simulink model "Test_21"  (R2024b)
settings: Solver=FixedStepAuto  StartTime=0.0  StopTime=50  RelTol=1e-3
undefined symbols (not defined in the file): BOOL, DINT, OTL, slplc
libraries: arduinolib x4
(part 9 of 10)

== matlab function Test_21/PLC Controller Suite/__Logic/Task/Program/__Logic/XIC1/__Format ==
  data: BlockEnable input; RungIn input; RungOut input; data input
function setBlockFormat(BlockEnable, RungIn, RungOut, data)

if data~=0 && data~=1
    error('slplc:inivalidBooleanValue', 'Invalid boolean value %d', data);
end
data = logical(data);

% set parent block colors
coder.extrinsic('slplc.utils.setBlockAppearance');
persistent lastBlockEnable lastRungIn lastRungOut lastData isInit lastAnimation lastDataShow;
if isempty(lastBlockEnable)
    lastBlockEnable = true;
end
if isempty(lastRungIn)
    lastRungIn = false;
end
if isempty(lastRungOut)
    lastRungOut = false;
end
if isempty(lastData)
    lastData = data;
end
if isempty(isInit)
    isInit = true;
else
    isInit = false;
end
if isempty(lastAnimation)
    lastAnimation = false;
end
if isempty(lastDataShow)
    lastDataShow = false;
end

[animation, dataShow] = slplc.utils.setBlockAppearance('set', '%<PLCOperandTag>', {}, {}, ...
    ' = ', {'ForegroundColor'}, ...
    isInit,  ...
    BlockEnable, lastBlockEnable, ...
    RungIn,  lastRungIn, ...
    RungOut, lastRungOut, ...
    data, lastData, ...
    lastAnimation, lastDataShow);

lastBlockEnable = BlockEnable;
lastRungIn      = RungIn;
lastRungOut     = RungOut;
lastData        = data;
lastAnimation   = animation;
lastDataShow    = dataShow;
end

== matlab function Test_21/PLC Controller Suite/__Logic/Task/Program/__Logic/Junction/__Format ==
  data: BlockEnable input; RungOut input
function setBlockFormat(BlockEnable, RungOut)
% set parent block colors
coder.extrinsic('slplc.utils.setBlockAppearance');
persistent lastBlockEnable isInit lastRungOut lastAnimation lastRungOutShow;
if isempty(lastBlockEnable)
    lastBlockEnable = true;
end

if isempty(isInit)
    isInit = true;
else
    isInit = false;
end

if isempty(lastRungOut)
    lastRungOut = RungOut;
end

if isempty(lastAnimation)
    lastAnimation = false;
end

if isempty(lastRungOutShow)
    lastRungOutShow = false;
end

[animation, dataShow] = slplc.utils.setBlockAppearance('set', '', {'black', 'black'}, {}, ...
    '', {'ForegroundColor', 'BackgroundColor'}, ...
    isInit,  ...
    BlockEnable, lastBlockEnable, ...
    RungOut,   lastRungOut, ...
    RungOut,   lastRungOut, ...
    [],    [], ...
    lastAnimation, lastRungOutShow);

lastBlockEnable     = BlockEnable;
lastRungOut         = RungOut;
lastAnimation       = animation;
lastRungOutShow     = dataShow;
end

== matlab function Test_21/PLC Controller Suite/__Logic/Task/Program/__Logic/OTL4/__Format ==
  data: BlockEnable input; RungIn input; RungOut input; data input
function setBlockFormat(BlockEnable, RungIn, RungOut, data)

if data~=0 && data~=1
    error('slplc:inivalidBooleanValue', 'Invalid boolean value %d', data);
end
data = logical(data);

% set parent block colors
coder.extrinsic('slplc.utils.setBlockAppearance');
persistent lastBlockEnable lastRungIn lastRungOut lastData isInit lastAnimation lastDataShow;
if isempty(lastBlockEnable)
    lastBlockEnable = true;
end
if isempty(lastRungIn)
    lastRungIn = false;
end
if isempty(lastRungOut)
    lastRungOut = false;
end
if isempty(lastData)
    lastData = data;
end
if isempty(isInit)
    isInit = true;
else
    isInit = false;
end
if isempty(lastAnimation)
    lastAnimation = false;
end
if isempty(lastDataShow)
    lastDataShow = false;
end

[animation, dataShow] = slplc.utils.setBlockAppearance('set', '%<PLCOperandTag>', {}, {}, ...
    ' = ', {'ForegroundColor'}, ...
    isInit,  ...
    BlockEnable, lastBlockEnable, ...
    RungIn,  lastRungIn, ...
    RungOut, lastRungOut, ...
    data, lastData, ...
    lastAnimation, lastDataShow);

lastBlockEnable = BlockEnable;
lastRungIn      = RungIn;
lastRungOut     = RungOut;
lastData        = data;
lastAnimation   = animation;
lastDataShow    = dataShow;
end

== matlab function Test_21/PLC Controller Suite/__Logic/Task/Program/__Logic/XIC3/__Format ==
  data: BlockEnable input; RungIn input; RungOut input; data input
function setBlockFormat(BlockEnable, RungIn, RungOut, data)

if data~=0 && data~=1
    error('slplc:inivalidBooleanValue', 'Invalid boolean value %d', data);
end
data = logical(data);

% set parent block colors
coder.extrinsic('slplc.utils.setBlockAppearance');
persistent lastBlockEnable lastRungIn lastRungOut lastData isInit lastAnimation lastDataShow;
if isempty(lastBlockEnable)
    lastBlockEnable = true;
end
if isempty(lastRungIn)
    lastRungIn = false;
end
if isempty(lastRungOut)
    lastRungOut = false;
end
if isempty(lastData)
    lastData = data;
end
if isempty(isInit)
    isInit = true;
else
    isInit = false;
end
if isempty(lastAnimation)
    lastAnimation = false;
end
if isempty(lastDataShow)
    lastDataShow = false;
end

[animation, dataShow] = slplc.utils.setBlockAppearance('set', '%<PLCOperandTag>', {}, {}, ...
    ' = ', {'ForegroundColor'}, ...
    isInit,  ...
    BlockEnable, lastBlockEnable, ...
    RungIn,  lastRungIn, ...
    RungOut, lastRungOut, ...
    data, lastData, ...
    lastAnimation, lastDataShow);

lastBlockEnable = BlockEnable;
lastRungIn      = RungIn;
lastRungOut     = RungOut;
lastData        = data;
lastAnimation   = animation;
lastDataShow    = dataShow;
end

== matlab function Test_21/PLC Controller Suite/__Logic/Task/Program/__Logic/OTL1/__Format ==
  data: BlockEnable input; RungIn input; RungOut input; data input
function setBlockFormat(BlockEnable, RungIn, RungOut, data)

if data~=0 && data~=1
    error('slplc:inivalidBooleanValue', 'Invalid boolean value %d', data);
end
data = logical(data);

% set parent block colors
coder.extrinsic('slplc.utils.setBlockAppearance');
persistent lastBlockEnable lastRungIn lastRungOut lastData isInit lastAnimation lastDataShow;
if isempty(lastBlockEnable)
    lastBlockEnable = true;
end
if isempty(lastRungIn)
    lastRungIn = false;
end
if isempty(lastRungOut)
    lastRungOut = false;
end
if isempty(lastData)
    lastData = data;
end
if isempty(isInit)
    isInit = true;
else
    isInit = false;
end
if isempty(lastAnimation)
    lastAnimation = false;
end
if isempty(lastDataShow)
    lastDataShow = false;
end

[animation, dataShow] = slplc.utils.setBlockAppearance('set', '%<PLCOperandTag>', {}, {}, ...
    ' = ', {'ForegroundColor'}, ...
    isInit,  ...
    BlockEnable, lastBlockEnable, ...
    RungIn,  lastRungIn, ...
    RungOut, lastRungOut, ...
    data, lastData, ...
    lastAnimation, lastDataShow);

lastBlockEnable = BlockEnable;
lastRungIn      = RungIn;
lastRungOut     = RungOut;
lastData        = data;
lastAnimation   = animation;
lastDataShow    = dataShow;
end

== matlab function Test_21/PLC Controller Suite/__Logic/Task/Program/__Logic/OTU9/__Format ==
  data: BlockEnable input; RungIn input; RungOut input; data input
function setBlockFormat(BlockEnable, RungIn, RungOut, data)

if data~=0 && data~=1
    error('slplc:inivalidBooleanValue', 'Invalid boolean value %d', data);
end
data = logical(data);

% set parent block colors
coder.extrinsic('slplc.utils.setBlockAppearance');
persistent lastBlockEnable lastRungIn lastRungOut lastData isInit lastAnimation lastDataShow;
if isempty(lastBlockEnable)
    lastBlockEnable = true;
end
if isempty(lastRungIn)
    lastRungIn = false;
end
if isempty(lastRungOut)
    lastRungOut = false;
end
if isempty(lastData)
    lastData = data;
end
if isempty(isInit)
    isInit = true;
else
    isInit = false;
end
if isempty(lastAnimation)
    lastAnimation = false;
end
if isempty(lastDataShow)
    lastDataShow = false;
end

[animation, dataShow] = slplc.utils.setBlockAppearance('set', '%<PLCOperandTag>', {}, {}, ...
    ' = ', {'ForegroundColor'}, ...
    isInit,  ...
    BlockEnable, lastBlockEnable, ...
    RungIn,  lastRungIn, ...
    RungOut, lastRungOut, ...
    data, lastData, ...
    lastAnimation, lastDataShow);

lastBlockEnable = BlockEnable;
lastRungIn      = RungIn;
lastRungOut     = RungOut;
lastData        = data;
lastAnimation   = animation;
lastDataShow    = dataShow;
end

== matlab function Test_21/PLC Controller Suite/__Logic/Task/Program/__Logic/OTU3/__Format ==
  data: BlockEnable input; RungIn input; RungOut input; data input
function setBlockFormat(BlockEnable, RungIn, RungOut, data)

if data~=0 && data~=1
    error('slplc:inivalidBooleanValue', 'Invalid boolean value %d', data);
end
data = logical(data);

% set parent block colors
coder.extrinsic('slplc.utils.setBlockAppearance');
persistent lastBlockEnable lastRungIn lastRungOut lastData isInit lastAnimation lastDataShow;
if isempty(lastBlockEnable)
    lastBlockEnable = true;
end
if isempty(lastRungIn)
    lastRungIn = false;
end
if isempty(lastRungOut)
    lastRungOut = false;
end
if isempty(lastData)
    lastData = data;
end
if isempty(isInit)
    isInit = true;
else
    isInit = false;
end
if isempty(lastAnimation)
    lastAnimation = false;
end
if isempty(lastDataShow)
    lastDataShow = false;
end

[animation, dataShow] = slplc.utils.setBlockAppearance('set', '%<PLCOperandTag>', {}, {}, ...
    ' = ', {'ForegroundColor'}, ...
    isInit,  ...
    BlockEnable, lastBlockEnable, ...
    RungIn,  lastRungIn, ...
    RungOut, lastRungOut, ...
    data, lastData, ...
    lastAnimation, lastDataShow);

lastBlockEnable = BlockEnable;
lastRungIn      = RungIn;
lastRungOut     = RungOut;
lastData        = data;
lastAnimation   = animation;
lastDataShow    = dataShow;
end

== matlab function Test_21/PLC Controller Suite/__Logic/Task/Program/__Logic/OTU4/__Format ==
  data: BlockEnable input; RungIn input; RungOut input; data input
function setBlockFormat(BlockEnable, RungIn, RungOut, data)

if data~=0 && data~=1
    error('slplc:inivalidBooleanValue', 'Invalid boolean value %d', data);
end
data = logical(data);

% set parent block colors
coder.extrinsic('slplc.utils.setBlockAppearance');
persistent lastBlockEnable lastRungIn lastRungOut lastData isInit lastAnimation lastDataShow;
if isempty(lastBlockEnable)
    lastBlockEnable = true;
end
if isempty(lastRungIn)
    lastRungIn = false;
end
if isempty(lastRungOut)
    lastRungOut = false;
end
if isempty(lastData)
    lastData = data;
end
if isempty(isInit)
    isInit = true;
else
    isInit = false;
end
if isempty(lastAnimation)
    lastAnimation = false;
end
if isempty(lastDataShow)
    lastDataShow = false;
end

[animation, dataShow] = slplc.utils.setBlockAppearance('set', '%<PLCOperandTag>', {}, {}, ...
    ' = ', {'ForegroundColor'}, ...
    isInit,  ...
    BlockEnable, lastBlockEnable, ...
    RungIn,  lastRungIn, ...
    RungOut, lastRungOut, ...
    data, lastData, ...
    lastAnimation, lastDataShow);

lastBlockEnable = BlockEnable;
lastRungIn      = RungIn;
lastRungOut     = RungOut;
lastData        = data;
lastAnimation   = animation;
lastDataShow    = dataShow;
end

== matlab function Test_21/PLC Controller Suite/__Logic/Task/Program/__Logic/OTL7/__Format ==
  data: BlockEnable input; RungIn input; RungOut input; data input
function setBlockFormat(BlockEnable, RungIn, RungOut, data)

if data~=0 && data~=1
    error('slplc:inivalidBooleanValue', 'Invalid boolean value %d', data);
end
data = logical(data);

% set parent block colors
coder.extrinsic('slplc.utils.setBlockAppearance');
persistent lastBlockEnable lastRungIn lastRungOut lastData isInit lastAnimation lastDataShow;
if isempty(lastBlockEnable)
    lastBlockEnable = true;
end
if isempty(lastRungIn)
    lastRungIn = false;
end
if isempty(lastRungOut)
    lastRungOut = false;
end
if isempty(lastData)
    lastData = data;
end
if isempty(isInit)
    isInit = true;
else
    isInit = false;
end
if isempty(lastAnimation)
    lastAnimation = false;
end
if isempty(lastDataShow)
    lastDataShow = false;
end

[animation, dataShow] = slplc.utils.setBlockAppearance('set', '%<PLCOperandTag>', {}, {}, ...
    ' = ', {'ForegroundColor'}, ...
    isInit,  ...
    BlockEnable, lastBlockEnable, ...
    RungIn,  lastRungIn, ...
    RungOut, lastRungOut, ...
    data, lastData, ...
    lastAnimation, lastDataShow);

lastBlockEnable = BlockEnable;
lastRungIn      = RungIn;
lastRungOut     = RungOut;
lastData        = data;
lastAnimation   = animation;
lastDataShow    = dataShow;
end

== matlab function Test_21/PLC Controller Suite/__Logic/Task/Program/__Logic/TON/Instruction_Enable/__Logic ==
  data: EN output; TT output; RungIn input; PRE input; EN input; DN input; DN output; ACC output; ACC input; currentTime input; lastTime input
function [EN, TT, DN, ACC]  = TON(RungIn, PRE, EN, DN, ACC, currentTime, lastTime)
% TON algorithm

if RungIn
    % Rung-condition-in is True
    if PRE < 0 || ACC < 0
        error('slplc:TONError', '.PRE or .ACC cannot be negtive values');
    end
    TT = true;
    if ~DN
        if EN
            deltaT = currentTime - lastTime;
            ACC = ACC + cast(deltaT, class(ACC));
            if ACC == intmax(class(ACC)) || ACC >= PRE
                TT = false;
                DN = true;
            end
        end
    else
        TT = false;
    end
    EN = true;
    % True end
else
    % Rung-condition-in is False
    EN    = false;
    TT    = false;
    DN    = false;
    ACC   = cast(0, class(ACC));
    % False end
end

end

== matlab function Test_21/PLC Controller Suite/__Logic/Task/Program/__Logic/XIC10/__Format ==
  data: BlockEnable input; RungIn input; RungOut input; data input
function setBlockFormat(BlockEnable, RungIn, RungOut, data)

if data~=0 && data~=1
    error('slplc:inivalidBooleanValue', 'Invalid boolean value %d', data);
end
data = logical(data);

% set parent block colors
coder.extrinsic('slplc.utils.setBlockAppearance');
persistent lastBlockEnable lastRungIn lastRungOut lastData isInit lastAnimation lastDataShow;
if isempty(lastBlockEnable)
    lastBlockEnable = true;
end
if isempty(lastRungIn)
    lastRungIn = false;
end
if isempty(lastRungOut)
    lastRungOut = false;
end
if isempty(lastData)
    lastData = data;
end
if isempty(isInit)
    isInit = true;
else
    isInit = false;
end
if isempty(lastAnimation)
    lastAnimation = false;
end
if isempty(lastDataShow)
    lastDataShow = false;
end

[animation, dataShow] = slplc.utils.setBlockAppearance('set', '%<PLCOperandTag>', {}, {}, ...
    ' = ', {'ForegroundColor'}, ...
    isInit,  ...
    BlockEnable, lastBlockEnable, ...
    RungIn,  lastRungIn, ...
    RungOut, lastRungOut, ...
    data, lastData, ...
    lastAnimation, lastDataShow);

lastBlockEnable = BlockEnable;
lastRungIn      = RungIn;
lastRungOut     = RungOut;
lastData        = data;
lastAnimation   = animation;
lastDataShow    = dataShow;
end

== matlab function Test_21/PLC Controller Suite/__Logic/Task/Program/__Logic/OTU2/__Format ==
  data: BlockEnable input; RungIn input; RungOut input; data input
function setBlockFormat(BlockEnable, RungIn, RungOut, data)

if data~=0 && data~=1
    error('slplc:inivalidBooleanValue', 'Invalid boolean value %d', data);
end
data = logical(data);

% set parent block colors
coder.extrinsic('slplc.utils.setBlockAppearance');
persistent lastBlockEnable lastRungIn lastRungOut lastData isInit lastAnimation lastDataShow;
if isempty(lastBlockEnable)
    lastBlockEnable = true;
end
if isempty(lastRungIn)
    lastRungIn = false;
end
if isempty(lastRungOut)
    lastRungOut = false;
end
if isempty(lastData)
    lastData = data;
end
if isempty(isInit)
    isInit = true;
else
    isInit = false;
end
if isempty(lastAnimation)
    lastAnimation = false;
end
if isempty(lastDataShow)
    lastDataShow = false;
end

[animation, dataShow] = slplc.utils.setBlockAppearance('set', '%<PLCOperandTag>', {}, {}, ...
    ' = ', {'ForegroundColor'}, ...
    isInit,  ...
    BlockEnable, lastBlockEnable, ...
    RungIn,  lastRungIn, ...
    RungOut, lastRungOut, ...
    data, lastData, ...
    lastAnimation, lastDataShow);

lastBlockEnable = BlockEnable;
lastRungIn      = RungIn;
lastRungOut     = RungOut;
lastData        = data;
lastAnimation   = animation;
lastDataShow    = dataShow;
end

== matlab function Test_21/PLC Controller Suite/__Logic/Task/Program/__Logic/XIO/__Format ==
  data: BlockEnable input; RungIn input; RungOut input; data input
function setBlockFormat(BlockEnable, RungIn, RungOut, data)

if data~=0 && data~=1
    error('slplc:inivalidBooleanValue', 'Invalid boolean value %d', data);
end
data = logical(data);

% set parent block colors
coder.extrinsic('slplc.utils.setBlockAppearance');
persistent lastBlockEnable lastRungIn lastRungOut lastData isInit lastAnimation lastDataShow;
if isempty(lastBlockEnable)
    lastBlockEnable = true;
end
if isempty(lastRungIn)
    lastRungIn = false;
end
if isempty(lastRungOut)
    lastRungOut = false;
end
if isempty(lastData)
    lastData = data;
end
if isempty(isInit)
    isInit = true;
else
    isInit = false;
end
if isempty(lastAnimation)
    lastAnimation = false;
end
if isempty(lastDataShow)
    lastDataShow = false;
end

[animation, dataShow] = slplc.utils.setBlockAppearance('set', '%<PLCOperandTag>', {}, {}, ...
    ' = ', {'ForegroundColor'}, ...
    isInit,  ...
    BlockEnable, lastBlockEnable, ...
    RungIn,  lastRungIn, ...
    RungOut, lastRungOut, ...
    data, lastData, ...
    lastAnimation, lastDataShow);

lastBlockEnable = BlockEnable;
lastRungIn      = RungIn;
lastRungOut     = RungOut;
lastData        = data;
lastAnimation   = animation;
lastDataShow    = dataShow;
end

== matlab function Test_21/PLC Controller Suite/__Logic/Task/Program/__Logic/XIC8/__Format ==
  data: BlockEnable input; RungIn input; RungOut input; data input
function setBlockFormat(BlockEnable, RungIn, RungOut, data)

if data~=0 && data~=1
    error('slplc:inivalidBooleanValue', 'Invalid boolean value %d', data);
end
data = logical(data);

% set parent block colors
coder.extrinsic('slplc.utils.setBlockAppearance');
persistent lastBlockEnable lastRungIn lastRungOut lastData isInit lastAnimation lastDataShow;
if isempty(lastBlockEnable)
    lastBlockEnable = true;
end
if isempty(lastRungIn)
    lastRungIn = false;
end
if isempty(lastRungOut)
    lastRungOut = false;
end
if isempty(lastData)
    lastData = data;
end
if isempty(isInit)
    isInit = true;
else
    isInit = false;
end
if isempty(lastAnimation)
    lastAnimation = false;
end
if isempty(lastDataShow)
    lastDataShow = false;
end

[animation, dataShow] = slplc.utils.setBlockAppearance('set', '%<PLCOperandTag>', {}, {}, ...
    ' = ', {'ForegroundColor'}, ...
    isInit,  ...
    BlockEnable, lastBlockEnable, ...
    RungIn,  lastRungIn, ...
    RungOut, lastRungOut, ...
    data, lastData, ...
    lastAnimation, lastDataShow);

lastBlockEnable = BlockEnable;
lastRungIn      = RungIn;
lastRungOut     = RungOut;
lastData        = data;
lastAnimation   = animation;
lastDataShow    = dataShow;
end

== matlab function Test_21/PLC Controller Suite/__Logic/Task/Program/__Logic/XIC6/__Format ==
  data: BlockEnable input; RungIn input; RungOut input; data input
function setBlockFormat(BlockEnable, RungIn, RungOut, data)

if data~=0 && data~=1
    error('slplc:inivalidBooleanValue', 'Invalid boolean value %d', data);
end
data = logical(data);

% set parent block colors
coder.extrinsic('slplc.utils.setBlockAppearance');
persistent lastBlockEnable lastRungIn lastRungOut lastData isInit lastAnimation lastDataShow;
if isempty(lastBlockEnable)
    lastBlockEnable = true;
end
if isempty(lastRungIn)
    lastRungIn = false;
end
if isempty(lastRungOut)
    lastRungOut = false;
end
if isempty(lastData)
    lastData = data;
end
if isempty(isInit)
    isInit = true;
else
    isInit = false;
end
if isempty(lastAnimation)
    lastAnimation = false;
end
if isempty(lastDataShow)
    lastDataShow = false;
end

[animation, dataShow] = slplc.utils.setBlockAppearance('set', '%<PLCOperandTag>', {}, {}, ...
    ' = ', {'ForegroundColor'}, ...
    isInit,  ...
    BlockEnable, lastBlockEnable, ...
    RungIn,  lastRungIn, ...
    RungOut, lastRungOut, ...
    data, lastData, ...
    lastAnimation, lastDataShow);

lastBlockEnable = BlockEnable;
lastRungIn      = RungIn;
lastRungOut     = RungOut;
lastData        = data;
lastAnimation   = animation;
lastDataShow    = dataShow;
end

== matlab function Test_21/PLC Controller Suite/__Logic/Task/Program/__Logic/OTU10/__Format ==
  data: BlockEnable input; RungIn input; RungOut input; data input
function setBlockFormat(BlockEnable, RungIn, RungOut, data)

if data~=0 && data~=1
    error('slplc:inivalidBooleanValue', 'Invalid boolean value %d', data);
end
data = logical(data);

% set parent block colors
coder.extrinsic('slplc.utils.setBlockAppearance');
persistent lastBlockEnable lastRungIn lastRungOut lastData isInit lastAnimation lastDataShow;
if isempty(lastBlockEnable)
    lastBlockEnable = true;
end
if isempty(lastRungIn)
    lastRungIn = false;
end
if isempty(lastRungOut)
    lastRungOut = false;
end
if isempty(lastData)
    lastData = data;
end
if isempty(isInit)
    isInit = true;
else
    isInit = false;
end
if isempty(lastAnimation)
    lastAnimation = false;
end
if isempty(lastDataShow)
    lastDataShow = false;
end

[animation, dataShow] = slplc.utils.setBlockAppearance('set', '%<PLCOperandTag>', {}, {}, ...
    ' = ', {'ForegroundColor'}, ...
    isInit,  ...
    BlockEnable, lastBlockEnable, ...
    RungIn,  lastRungIn, ...
    RungOut, lastRungOut, ...
    data, lastData, ...
    lastAnimation, lastDataShow);

lastBlockEnable = BlockEnable;
lastRungIn      = RungIn;
lastRungOut     = RungOut;
lastData        = data;
lastAnimation   = animation;
lastDataShow    = dataShow;
end

== matlab function Test_21/PLC Controller Suite/__Logic/Task/Program/__Logic/OTL2/__Format ==
  data: BlockEnable input; RungIn input; RungOut input; data input
function setBlockFormat(BlockEnable, RungIn, RungOut, data)

if data~=0 && data~=1
    error('slplc:inivalidBooleanValue', 'Invalid boolean value %d', data);
end
data = logical(data);

% set parent block colors
coder.extrinsic('slplc.utils.setBlockAppearance');
persistent lastBlockEnable lastRungIn lastRungOut lastData isInit lastAnimation lastDataShow;
if isempty(lastBlockEnable)
    lastBlockEnable = true;
end
if isempty(lastRungIn)
    lastRungIn = false;
end
if isempty(lastRungOut)
    lastRungOut = false;
end
if isempty(lastData)
    lastData = data;
end
if isempty(isInit)
    isInit = true;
else
    isInit = false;
end
if isempty(lastAnimation)
    lastAnimation = false;
end
if isempty(lastDataShow)
    lastDataShow = false;
end

[animation, dataShow] = slplc.utils.setBlockAppearance('set', '%<PLCOperandTag>', {}, {}, ...
    ' = ', {'ForegroundColor'}, ...
    isInit,  ...
    BlockEnable, lastBlockEnable, ...
    RungIn,  lastRungIn, ...
    RungOut, lastRungOut, ...
    data, lastData, ...
    lastAnimation, lastDataShow);

lastBlockEnable = BlockEnable;
lastRungIn      = RungIn;
lastRungOut     = RungOut;
lastData        = data;
lastAnimation   = animation;
lastDataShow    = dataShow;
end

== matlab function Test_21/PLC Controller Suite/__Logic/Task/Program/__Logic/OTU/__Format ==
  data: BlockEnable input; RungIn input; RungOut input; data input
function setBlockFormat(BlockEnable, RungIn, RungOut, data)

if data~=0 && data~=1
    error('slplc:inivalidBooleanValue', 'Invalid boolean value %d', data);
end
data = logical(data);

% set parent block colors
coder.extrinsic('slplc.utils.setBlockAppearance');
persistent lastBlockEnable lastRungIn lastRungOut lastData isInit lastAnimation lastDataShow;
if isempty(lastBlockEnable)
    lastBlockEnable = true;
end
if isempty(lastRungIn)
    lastRungIn = false;
end
if isempty(lastRungOut)
    lastRungOut = false;
end
if isempty(lastData)
    lastData = data;
end
if isempty(isInit)
    isInit = true;
else
    isInit = false;
end
if isempty(lastAnimation)
    lastAnimation = false;
end
if isempty(lastDataShow)
    lastDataShow = false;
end

[animation, dataShow] = slplc.utils.setBlockAppearance('set', '%<PLCOperandTag>', {}, {}, ...
    ' = ', {'ForegroundColor'}, ...
    isInit,  ...
    BlockEnable, lastBlockEnable, ...
    RungIn,  lastRungIn, ...
    RungOut, lastRungOut, ...
    data, lastData, ...
    lastAnimation, lastDataShow);

lastBlockEnable = BlockEnable;
lastRungIn      = RungIn;
lastRungOut     = RungOut;
lastData        = data;
lastAnimation   = animation;
lastDataShow    = dataShow;
end

== matlab function Test_21/PLC Controller Suite/__Logic/Task/Program/__Logic/OTU1/__Format ==
  data: BlockEnable input; RungIn input; RungOut input; data input
function setBlockFormat(BlockEnable, RungIn, RungOut, data)

if data~=0 && data~=1
    error('slplc:inivalidBooleanValue', 'Invalid boolean value %d', data);
end
data = logical(data);

% set parent block colors
coder.extrinsic('slplc.utils.setBlockAppearance');
persistent lastBlockEnable lastRungIn lastRungOut lastData isInit lastAnimation lastDataShow;
if isempty(lastBlockEnable)
    lastBlockEnable = true;
end
if isempty(lastRungIn)
    lastRungIn = false;
end
if isempty(lastRungOut)
    lastRungOut = false;
end
if isempty(lastData)
    lastData = data;
end
if isempty(isInit)
    isInit = true;
else
    isInit = false;
end
if isempty(lastAnimation)
    lastAnimation = false;
end
if isempty(lastDataShow)
    lastDataShow = false;
end

[animation, dataShow] = slplc.utils.setBlockAppearance('set', '%<PLCOperandTag>', {}, {}, ...
    ' = ', {'ForegroundColor'}, ...
    isInit,  ...
    BlockEnable, lastBlockEnable, ...
    RungIn,  lastRungIn, ...
    RungOut, lastRungOut, ...
    data, lastData, ...
    lastAnimation, lastDataShow);

lastBlockEnable = BlockEnable;
lastRungIn      = RungIn;
lastRungOut     = RungOut;
lastData        = data;
lastAnimation   = animation;
lastDataShow    = dataShow;
end

== matlab function Test_21/PLC Controller Suite/__Logic/Task/Program/__Logic/XIO3/__Format ==
  data: BlockEnable input; RungIn input; RungOut input; data input
function setBlockFormat(BlockEnable, RungIn, RungOut, data)

if data~=0 && data~=1
    error('slplc:inivalidBooleanValue', 'Invalid boolean value %d', data);
end
data = logical(data);

% set parent block colors
coder.extrinsic('slplc.utils.setBlockAppearance');
persistent lastBlockEnable lastRungIn lastRungOut lastData isInit lastAnimation lastDataShow;
if isempty(lastBlockEnable)
    lastBlockEnable = true;
end
if isempty(lastRungIn)
    lastRungIn = false;
end
if isempty(lastRungOut)
    lastRungOut = false;
end
if isempty(lastData)
    lastData = data;
end
if isempty(isInit)
    isInit = true;
else
    isInit = false;
end
if isempty(lastAnimation)
    lastAnimation = false;
end
if isempty(lastDataShow)
    lastDataShow = false;
end

[animation, dataShow] = slplc.utils.setBlockAppearance('set', '%<PLCOperandTag>', {}, {}, ...
    ' = ', {'ForegroundColor'}, ...
    isInit,  ...
    BlockEnable, lastBlockEnable, ...
    RungIn,  lastRungIn, ...
    RungOut, lastRungOut, ...
    data, lastData, ...
    lastAnimation, lastDataShow);

lastBlockEnable = BlockEnable;
lastRungIn      = RungIn;
lastRungOut     = RungOut;
lastData        = data;
lastAnimation   = animation;
lastDataShow    = dataShow;
end

== matlab function Test_21/PLC Controller Suite/__Logic/Task/Program/__Logic/OTU5/__Format ==
  data: BlockEnable input; RungIn input; RungOut input; data input
function setBlockFormat(BlockEnable, RungIn, RungOut, data)

if data~=0 && data~=1
    error('slplc:inivalidBooleanValue', 'Invalid boolean value %d', data);
end
data = logical(data);

% set parent block colors
coder.extrinsic('slplc.utils.setBlockAppearance');
persistent lastBlockEnable lastRungIn lastRungOut lastData isInit lastAnimation lastDataShow;
if isempty(lastBlockEnable)
    lastBlockEnable = true;
end
if isempty(lastRungIn)
    lastRungIn = false;
end
if isempty(lastRungOut)
    lastRungOut = false;
end
if isempty(lastData)
    lastData = data;
end
if isempty(isInit)
    isInit = true;
else
    isInit = false;
end
if isempty(lastAnimation)
    lastAnimation = false;
end
if isempty(lastDataShow)
    lastDataShow = false;
end

[animation, dataShow] = slplc.utils.setBlockAppearance('set', '%<PLCOperandTag>', {}, {}, ...
    ' = ', {'ForegroundColor'}, ...
    isInit,  ...
    BlockEnable, lastBlockEnable, ...
    RungIn,  lastRungIn, ...
    RungOut, lastRungOut, ...
    data, lastData, ...
    lastAnimation, lastDataShow);

lastBlockEnable = BlockEnable;
lastRungIn      = RungIn;
lastRungOut     = RungOut;
lastData        = data;
lastAnimation   = animation;
lastDataShow    = dataShow;
end

== matlab function Test_21/PLC Controller Suite/__Logic/Task/Program/__Logic/XIC7/__Format ==
  data: BlockEnable input; RungIn input; RungOut input; data input
function setBlockFormat(BlockEnable, RungIn, RungOut, data)

if data~=0 && data~=1
    error('slplc:inivalidBooleanValue', 'Invalid boolean value %d', data);
end
data = logical(data);

% set parent block colors
coder.extrinsic('slplc.utils.setBlockAppearance');
persistent lastBlockEnable lastRungIn lastRungOut lastData isInit lastAnimation lastDataShow;
if isempty(lastBlockEnable)
    lastBlockEnable = true;
end
if isempty(lastRungIn)
    lastRungIn = false;
end
if isempty(lastRungOut)
    lastRungOut = false;
end
if isempty(lastData)
    lastData = data;
end
if isempty(isInit)
    isInit = true;
else
    isInit = false;
end
if isempty(lastAnimation)
    lastAnimation = false;
end
if isempty(lastDataShow)
    lastDataShow = false;
end

[animation, dataShow] = slplc.utils.setBlockAppearance('set', '%<PLCOperandTag>', {}, {}, ...
    ' = ', {'ForegroundColor'}, ...
    isInit,  ...
    BlockEnable, lastBlockEnable, ...
    RungIn,  lastRungIn, ...
    RungOut, lastRungOut, ...
    data, lastData, ...
    lastAnimation, lastDataShow);

lastBlockEnable = BlockEnable;
lastRungIn      = RungIn;
lastRungOut     = RungOut;
lastData        = data;
lastAnimation   = animation;
lastDataShow    = dataShow;
end

== matlab function Test_21/PLC Controller Suite/__Logic/Task/Program/__Logic/XIO2/__Format ==
  data: BlockEnable input; RungIn input; RungOut input; data input
function setBlockFormat(BlockEnable, RungIn, RungOut, data)

if data~=0 && data~=1
    error('slplc:inivalidBooleanValue', 'Invalid boolean value %d', data);
end
data = logical(data);

% set parent block colors
coder.extrinsic('slplc.utils.setBlockAppearance');
persistent lastBlockEnable lastRungIn lastRungOut lastData isInit lastAnimation lastDataShow;
if isempty(lastBlockEnable)
    lastBlockEnable = true;
end
if isempty(lastRungIn)
    lastRungIn = false;
end
if isempty(lastRungOut)
    lastRungOut = false;
end
if isempty(lastData)
    lastData = data;
end
if isempty(isInit)
    isInit = true;
else
    isInit = false;
end
if isempty(lastAnimation)
    lastAnimation = false;
end
if isempty(lastDataShow)
    lastDataShow = false;
end

[animation, dataShow] = slplc.utils.setBlockAppearance('set', '%<PLCOperandTag>', {}, {}, ...
    ' = ', {'ForegroundColor'}, ...
    isInit,  ...
    BlockEnable, lastBlockEnable, ...
    RungIn,  lastRungIn, ...
    RungOut, lastRungOut, ...
    data, lastData, ...
    lastAnimation, lastDataShow);

lastBlockEnable = BlockEnable;
lastRungIn      = RungIn;
lastRungOut     = RungOut;
lastData        = data;
lastAnimation   = animation;
lastDataShow    = dataShow;
end

== matlab function Test_21/PLC Controller Suite/__Logic/Task/Program/__Logic/OTE3/__Format ==
  data: BlockEnable input; RungIn input; RungOut input; data input
function setBlockFormat(BlockEnable, RungIn, RungOut, data)

if data~=0 && data~=1
    error('slplc:inivalidBooleanValue', 'Invalid boolean value %d', data);
end
data = logical(data);

% set parent block colors
coder.extrinsic('slplc.utils.setBlockAppearance');
persistent lastBlockEnable lastRungIn lastRungOut lastData isInit lastAnimation lastDataShow;
if isempty(lastBlockEnable)
    lastBlockEnable = true;
end
if isempty(lastRungIn)
    lastRungIn = false;
end
if isempty(lastRungOut)
    lastRungOut = false;
end
if isempty(lastData)
    lastData = data;
end
if isempty(isInit)
    isInit = true;
else
    isInit = false;
end
if isempty(lastAnimation)
    lastAnimation = false;
end
if isempty(lastDataShow)
    lastDataShow = false;
end

[animation, dataShow] = slplc.utils.setBlockAppearance('set', '%<PLCOperandTag>', {}, {}, ...
    ' = ', {'ForegroundColor'}, ...
    isInit,  ...
    BlockEnable, lastBlockEnable, ...
    RungIn,  lastRungIn, ...
    RungOut, lastRungOut, ...
    data, lastData, ...
    lastAnimation, lastDataShow);

lastBlockEnable = BlockEnable;
lastRungIn      = RungIn;
lastRungOut     = RungOut;
lastData        = data;
lastAnimation   = animation;
lastDataShow    = dataShow;
end

== matlab function Test_21/PLC Controller Suite/__Logic/Task/Program/__Logic/TON3/Instruction_Enable/__Logic ==
  data: EN output; TT output; RungIn input; PRE input; EN input; DN input; DN output; ACC output; ACC input; currentTime input; lastTime input
function [EN, TT, DN, ACC]  = TON(RungIn, PRE, EN, DN, ACC, currentTime, lastTime)
% TON algorithm

if RungIn
    % Rung-condition-in is True
    if PRE < 0 || ACC < 0
        error('slplc:TONError', '.PRE or .ACC cannot be negtive values');
    end
    TT = true;
    if ~DN
        if EN
            deltaT = currentTime - lastTime;
            ACC = ACC + cast(deltaT, class(ACC));
            if ACC == intmax(class(ACC)) || ACC >= PRE
                TT = false;
                DN = true;
            end
        end
    else
        TT = false;
    end
    EN = true;
    % True end
else
    % Rung-condition-in is False
    EN    = false;
    TT    = false;
    DN    = false;
    ACC   = cast(0, class(ACC));
    % False end
end

end

== matlab function Test_21/PLC Controller Suite/__Logic/Task/Program/__Logic/TON3/__Format ==
  data: BlockEnable input; RungIn input; RungOut input; data input
function setBlockFormat(BlockEnable, RungIn, RungOut, data)
% set parent block colors
coder.extrinsic('slplc.utils.setBlockAppearance');
persistent lastBlockEnable lastRungIn lastRungOut lastData isInit lastAnimation lastDataShow;
if isempty(lastBlockEnable)
    lastBlockEnable = true;
end
if isempty(lastRungIn)
    lastRungIn = false;
end
if isempty(lastRungOut)
    lastRungOut = false;
end
if isempty(lastData)
    lastData = data;
end
if isempty(isInit)
    isInit = true;
else
    isInit = false;
end
if isempty(lastAnimation)
    lastAnimation = false;
end
if isempty(lastDataShow)
    lastDataShow = false;
end

[animation, dataShow] = slplc.utils.setBlockAppearance('set', '%<PLCBlockType>: %<PLCOperandTag>', {}, {}, ...
    ' = ', {'ForegroundColor'}, ...
    isInit,  ...
    BlockEnable, lastBlockEnable, ...
    RungIn,  lastRungIn, ...
    RungOut, lastRungOut, ...
    data, lastData, ...
    lastAnimation, lastDataShow);

lastBlockEnable = BlockEnable;
lastRungIn      = RungIn;
lastRungOut     = RungOut;
lastData        = data;
lastAnimation   = animation;
lastDataShow    = dataShow;
end

== matlab function Test_21/PLC Controller Suite/__Logic/Task/Program/__Logic/OTU6/__Format ==
  data: BlockEnable input; RungIn input; RungOut input; data input
function setBlockFormat(BlockEnable, RungIn, RungOut, data)

if data~=0 && data~=1
    error('slplc:inivalidBooleanValue', 'Invalid boolean value %d', data);
end
data = logical(data);

% set parent block colors
coder.extrinsic('slplc.utils.setBlockAppearance');
persistent lastBlockEnable lastRungIn lastRungOut lastData isInit lastAnimation lastDataShow;
if isempty(lastBlockEnable)
    lastBlockEnable = true;
end
if isempty(lastRungIn)
    lastRungIn = false;
end
if isempty(lastRungOut)
    lastRungOut = false;
end
if isempty(lastData)
    lastData = data;
end
if isempty(isInit)
    isInit = true;
else
    isInit = false;
end
if isempty(lastAnimation)
    lastAnimation = false;
end
if isempty(lastDataShow)
    lastDataShow = false;
end

[animation, dataShow] = slplc.utils.setBlockAppearance('set', '%<PLCOperandTag>', {}, {}, ...
    ' = ', {'ForegroundColor'}, ...
    isInit,  ...
    BlockEnable, lastBlockEnable, ...
    RungIn,  lastRungIn, ...
    RungOut, lastRungOut, ...
    data, lastData, ...
    lastAnimation, lastDataShow);

lastBlockEnable = BlockEnable;
lastRungIn      = RungIn;
lastRungOut     = RungOut;
lastData        = data;
lastAnimation   = animation;
lastDataShow    = dataShow;
end

== matlab function Test_21/PLC Controller Suite/__Logic/Task/Program/__Logic/XIC9/__Format ==
  data: BlockEnable input; RungIn input; RungOut input; data input
function setBlockFormat(BlockEnable, RungIn, RungOut, data)

if data~=0 && data~=1
    error('slplc:inivalidBooleanValue', 'Invalid boolean value %d', data);
end
data = logical(data);

% set parent block colors
coder.extrinsic('slplc.utils.setBlockAppearance');
persistent lastBlockEnable lastRungIn lastRungOut lastData isInit lastAnimation lastDataShow;
if isempty(lastBlockEnable)
    lastBlockEnable = true;
end
if isempty(lastRungIn)
    lastRungIn = false;
end
if isempty(lastRungOut)
    lastRungOut = false;
end
if isempty(lastData)
    lastData = data;
end
if isempty(isInit)
    isInit = true;
else
    isInit = false;
end
if isempty(lastAnimation)
    lastAnimation = false;
end
if isempty(lastDataShow)
    lastDataShow = false;
end

[animation, dataShow] = slplc.utils.setBlockAppearance('set', '%<PLCOperandTag>', {}, {}, ...
    ' = ', {'ForegroundColor'}, ...
    isInit,  ...
    BlockEnable, lastBlockEnable, ...
    RungIn,  lastRungIn, ...
    RungOut, lastRungOut, ...
    data, lastData, ...
    lastAnimation, lastDataShow);

lastBlockEnable = BlockEnable;
lastRungIn      = RungIn;
lastRungOut     = RungOut;
lastData        = data;
lastAnimation   = animation;
lastDataShow    = dataShow;
end

== matlab function Test_21/PLC Controller Suite/__Logic/Task/Program/__Logic/Junction1/__Format ==
  data: BlockEnable input; RungOut input
function setBlockFormat(BlockEnable, RungOut)
% set parent block colors
coder.extrinsic('slplc.utils.setBlockAppearance');
persistent lastBlockEnable isInit lastRungOut lastAnimation lastRungOutShow;
if isempty(lastBlockEnable)
    lastBlockEnable = true;
end

if isempty(isInit)
    isInit = true;
else
    isInit = false;
end

if isempty(lastRungOut)
    lastRungOut = RungOut;
end

if isempty(lastAnimation)
    lastAnimation = false;
end

if isempty(lastRungOutShow)
    lastRungOutShow = false;
end

[animation, dataShow] = slplc.utils.setBlockAppearance('set', '', {'black', 'black'}, {}, ...
    '', {'ForegroundColor', 'BackgroundColor'}, ...
    isInit,  ...
    BlockEnable, lastBlockEnable, ...
    RungOut,   lastRungOut, ...
    RungOut,   lastRungOut, ...
    [],    [], ...
    lastAnimation, lastRungOutShow);

lastBlockEnable     = BlockEnable;
lastRungOut         = RungOut;
lastAnimation       = animation;
lastRungOutShow     = dataShow;
end

== matlab function Test_21/PLC Controller Suite/__Logic/Task/Program/__Logic/OTU7/__Format ==
  data: BlockEnable input; RungIn input; RungOut input; data input
function setBlockFormat(BlockEnable, RungIn, RungOut, data)

if data~=0 && data~=1
    error('slplc:inivalidBooleanValue', 'Invalid boolean value %d', data);
end
data = logical(data);

% set parent block colors
coder.extrinsic('slplc.utils.setBlockAppearance');
persistent lastBlockEnable lastRungIn lastRungOut lastData isInit lastAnimation lastDataShow;
if isempty(lastBlockEnable)
    lastBlockEnable = true;
end
if isempty(lastRungIn)
    lastRungIn = false;
end
if isempty(lastRungOut)
    lastRungOut = false;
end
if isempty(lastData)
    lastData = data;
end
if isempty(isInit)
    isInit = true;
else
    isInit = false;
end
if isempty(lastAnimation)
    lastAnimation = false;
end
if isempty(lastDataShow)
    lastDataShow = false;
end

[animation, dataShow] = slplc.utils.setBlockAppearance('set', '%<PLCOperandTag>', {}, {}, ...
    ' = ', {'ForegroundColor'}, ...
    isInit,  ...
    BlockEnable, lastBlockEnable, ...
    RungIn,  lastRungIn, ...
    RungOut, lastRungOut, ...
    data, lastData, ...
    lastAnimation, lastDataShow);

lastBlockEnable = BlockEnable;
lastRungIn      = RungIn;
lastRungOut     = RungOut;
lastData        = data;
lastAnimation   = animation;
lastDataShow    = dataShow;
end

== matlab function Test_21/PLC Controller Suite/__Logic/Task/Program/__Logic/OTL5/__Format ==
  data: BlockEnable input; RungIn input; RungOut input; data input
function setBlockFormat(BlockEnable, RungIn, RungOut, data)

if data~=0 && data~=1
    error('slplc:inivalidBooleanValue', 'Invalid boolean value %d', data);
end
data = logical(data);

% set parent block colors
coder.extrinsic('slplc.utils.setBlockAppearance');
persistent lastBlockEnable lastRungIn lastRungOut lastData isInit lastAnimation lastDataShow;
if isempty(lastBlockEnable)
    lastBlockEnable = true;
end
if isempty(lastRungIn)
    lastRungIn = false;
end
if isempty(lastRungOut)
    lastRungOut = false;
end
if isempty(lastData)
    lastData = data;
end
if isempty(isInit)
    isInit = true;
else
    isInit = false;
end
if isempty(lastAnimation)
    lastAnimation = false;
end
if isempty(lastDataShow)
    lastDataShow = false;
end

[animation, dataShow] = slplc.utils.setBlockAppearance('set', '%<PLCOperandTag>', {}, {}, ...
    ' = ', {'ForegroundColor'}, ...
    isInit,  ...
    BlockEnable, lastBlockEnable, ...
    RungIn,  lastRungIn, ...
    RungOut, lastRungOut, ...
    data, lastData, ...
    lastAnimation, lastDataShow);

lastBlockEnable = BlockEnable;
lastRungIn      = RungIn;
lastRungOut     = RungOut;
lastData        = data;
lastAnimation   = animation;
lastDataShow    = dataShow;
end

== matlab function Test_21/PLC Controller Suite/__Logic/Task/Program/__Logic/OTL6/__Format ==
  data: BlockEnable input; RungIn input; RungOut input; data input
function setBlockFormat(BlockEnable, RungIn, RungOut, data)

if data~=0 && data~=1
    error('slplc:inivalidBooleanValue', 'Invalid boolean value %d', data);
end
data = logical(data);

% set parent block colors
coder.extrinsic('slplc.utils.setBlockAppearance');
persistent lastBlockEnable lastRungIn lastRungOut lastData isInit lastAnimation lastDataShow;
if isempty(lastBlockEnable)
    lastBlockEnable = true;
end
if isempty(lastRungIn)
    lastRungIn = false;
end
if isempty(lastRungOut)
    lastRungOut = false;
end
if isempty(lastData)
    lastData = data;
end
if isempty(isInit)
    isInit = true;
else
    isInit = false;
end
if isempty(lastAnimation)
    lastAnimation = false;
end
if isempty(lastDataShow)
    lastDataShow = false;
end

[animation, dataShow] = slplc.utils.setBlockAppearance('set', '%<PLCOperandTag>', {}, {}, ...
    ' = ', {'ForegroundColor'}, ...
    isInit,  ...
    BlockEnable, lastBlockEnable, ...
    RungIn,  lastRungIn, ...
    RungOut, lastRungOut, ...
    data, lastData, ...
    lastAnimation, lastDataShow);

lastBlockEnable = BlockEnable;
lastRungIn      = RungIn;
lastRungOut     = RungOut;
lastData        = data;
lastAnimation   = animation;
lastDataShow    = dataShow;
end

== matlab function Test_21/PLC Controller Suite/__Logic/Task/Program/__Logic/XIO1/__Format ==
  data: BlockEnable input; RungIn input; RungOut input; data input
function setBlockFormat(BlockEnable, RungIn, RungOut, data)

if data~=0 && data~=1
    error('slplc:inivalidBooleanValue', 'Invalid boolean value %d', data);
end
data = logical(data);

% set parent block colors
coder.extrinsic('slplc.utils.setBlockAppearance');
persistent lastBlockEnable lastRungIn lastRungOut lastData isInit lastAnimation lastDataShow;
if isempty(lastBlockEnable)
    lastBlockEnable = true;
end
if isempty(lastRungIn)
    lastRungIn = false;
end
if isempty(lastRungOut)
    lastRungOut = false;
end
if isempty(lastData)
    lastData = data;
end
if isempty(isInit)
    isInit = true;
else
    isInit = false;
end
if isempty(lastAnimation)
    lastAnimation = false;
end
if isempty(lastDataShow)
    lastDataShow = false;
end

[animation, dataShow] = slplc.utils.setBlockAppearance('set', '%<PLCOperandTag>', {}, {}, ...
    ' = ', {'ForegroundColor'}, ...
    isInit,  ...
    BlockEnable, lastBlockEnable, ...
    RungIn,  lastRungIn, ...
    RungOut, lastRungOut, ...
    data, lastData, ...
    lastAnimation, lastDataShow);

lastBlockEnable = BlockEnable;
lastRungIn      = RungIn;
lastRungOut     = RungOut;
lastData        = data;
lastAnimation   = animation;
lastDataShow    = dataShow;
end

== matlab function Test_21/PLC Controller Suite/__Logic/Task/Program/__Logic/OTU8/__Format ==
  data: BlockEnable input; RungIn input; RungOut input; data input
function setBlockFormat(BlockEnable, RungIn, RungOut, data)

if data~=0 && data~=1
    error('slplc:inivalidBooleanValue', 'Invalid boolean value %d', data);
end
data = logical(data);

% set parent block colors
coder.extrinsic('slplc.utils.setBlockAppearance');
persistent lastBlockEnable lastRungIn lastRungOut lastData isInit lastAnimation lastDataShow;
if isempty(lastBlockEnable)
    lastBlockEnable = true;
end
if isempty(lastRungIn)
    lastRungIn = false;
end
if isempty(lastRungOut)
    lastRungOut = false;
end
if isempty(lastData)
    lastData = data;
end
if isempty(isInit)
    isInit = true;
else
    isInit = false;
end
if isempty(lastAnimation)
    lastAnimation = false;
end
if isempty(lastDataShow)
    lastDataShow = false;
end

[animation, dataShow] = slplc.utils.setBlockAppearance('set', '%<PLCOperandTag>', {}, {}, ...
    ' = ', {'ForegroundColor'}, ...
    isInit,  ...
    BlockEnable, lastBlockEnable, ...
    RungIn,  lastRungIn, ...
    RungOut, lastRungOut, ...
    data, lastData, ...
    lastAnimation, lastDataShow);

lastBlockEnable = BlockEnable;
lastRungIn      = RungIn;
lastRungOut     = RungOut;
lastData        = data;
lastAnimation   = animation;
lastDataShow    = dataShow;
end

== matlab function Test_21/PLC Controller Suite/__Logic/Task/Program/__Logic/OTE4/__Format ==
  data: BlockEnable input; RungIn input; RungOut input; data input
function setBlockFormat(BlockEnable, RungIn, RungOut, data)

if data~=0 && data~=1
    error('slplc:inivalidBooleanValue', 'Invalid boolean value %d', data);
end
data = logical(data);

% set parent block colors
coder.extrinsic('slplc.utils.setBlockAppearance');
persistent lastBlockEnable lastRungIn lastRungOut lastData isInit lastAnimation lastDataShow;
if isempty(lastBlockEnable)
    lastBlockEnable = true;
end
if isempty(lastRungIn)
    lastRungIn = false;
end
if isempty(lastRungOut)
    lastRungOut = false;
end
if isempty(lastData)
    lastData = data;
end
if isempty(isInit)
    isInit = true;
else
    isInit = false;
end
if isempty(lastAnimation)
    lastAnimation = false;
end
if isempty(lastDataShow)
    lastDataShow = false;
end

[animation, dataShow] = slplc.utils.setBlockAppearance('set', '%<PLCOperandTag>', {}, {}, ...
    ' = ', {'ForegroundColor'}, ...
    isInit,  ...
    BlockEnable, lastBlockEnable, ...
    RungIn,  lastRungIn, ...
    RungOut, lastRungOut, ...
    data, lastData, ...
    lastAnimation, lastDataShow);

lastBlockEnable = BlockEnable;
lastRungIn      = RungIn;
lastRungOut     = RungOut;
lastData        = data;
lastAnimation   = animation;
lastDataShow    = dataShow;
end

== matlab function Test_21/PLC Controller Suite/__Logic/Task/Program/__Logic/TON4/Instruction_Enable/__Logic ==
  data: EN output; TT output; RungIn input; PRE input; EN input; DN input; DN output; ACC output; ACC input; currentTime input; lastTime input
function [EN, TT, DN, ACC]  = TON(RungIn, PRE, EN, DN, ACC, currentTime, lastTime)
% TON algorithm

if RungIn
    % Rung-condition-in is True
    if PRE < 0 || ACC < 0
        error('slplc:TONError', '.PRE or .ACC cannot be negtive values');
    end
    TT = true;
    if ~DN
        if EN
            deltaT = currentTime - lastTime;
            ACC = ACC + cast(deltaT, class(ACC));
            if ACC == intmax(class(ACC)) || ACC >= PRE
                TT = false;
                DN = true;
            end
        end
    else
        TT = false;
    end
    EN = true;
    % True end
else
    % Rung-condition-in is False
    EN    = false;
    TT    = false;
    DN    = false;
    ACC   = cast(0, class(ACC));
    % False end
end

end

== matlab function Test_21/PLC Controller Suite/__Logic/Task/Program/__Logic/OTL3/__Format ==
  data: BlockEnable input; RungIn input; RungOut input; data input
function setBlockFormat(BlockEnable, RungIn, RungOut, data)

if data~=0 && data~=1
    error('slplc:inivalidBooleanValue', 'Invalid boolean value %d', data);
end
data = logical(data);

% set parent block colors
coder.extrinsic('slplc.utils.setBlockAppearance');
persistent lastBlockEnable lastRungIn lastRungOut lastData isInit lastAnimation lastDataShow;
if isempty(lastBlockEnable)
    lastBlockEnable = true;
end
if isempty(lastRungIn)
    lastRungIn = false;
end
if isempty(lastRungOut)
    lastRungOut = false;
end
if isempty(lastData)
    lastData = data;
end
if isempty(isInit)
    isInit = true;
else
    isInit = false;
end
if isempty(lastAnimation)
    lastAnimation = false;
end
if isempty(lastDataShow)
    lastDataShow = false;
end

[animation, dataShow] = slplc.utils.setBlockAppearance('set', '%<PLCOperandTag>', {}, {}, ...
    ' = ', {'ForegroundColor'}, ...
    isInit,  ...
    BlockEnable, lastBlockEnable, ...
    RungIn,  lastRungIn, ...
    RungOut, lastRungOut, ...
    data, lastData, ...
    lastAnimation, lastDataShow);

lastBlockEnable = BlockEnable;
lastRungIn      = RungIn;
lastRungOut     = RungOut;
lastData        = data;
lastAnimation   = animation;
lastDataShow    = dataShow;
end
